simulink model "SIMULAZIONE_AF"  (R2020b)
settings: Solver=VariableStepAuto  StartTime=0.0  StopTime=10  RelTol=1e-3
libraries: simulink x1, dsparch4 x1
settings Model: Creator=danie  LastModifiedBy=danie

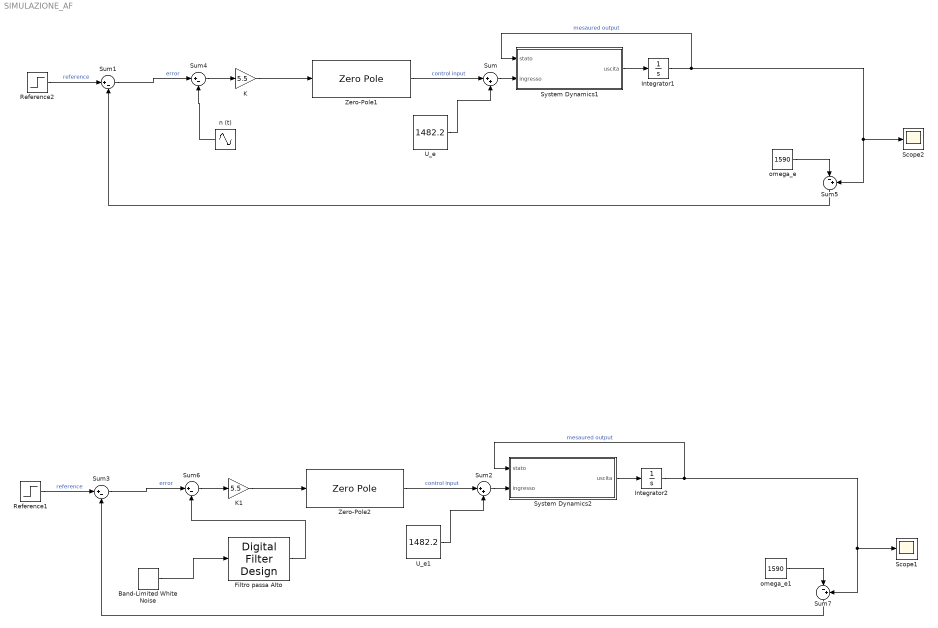
== system SIMULAZIONE_AF ==
  Band-Limited White Noise : simulink/Sources/Band-Limited White Noise  Cov=[500]  Ts=0.1  seed=[23341]
  Filtro passa Alto : dsparch4/Digital Filter Design  mwdsp_browser_bugfix_var=off
  Integrator1 : Integrator  InitialCondition=1590
  Integrator2 : Integrator  InitialCondition=1590
  K : Gain  Gain=5.5
  K1 : Gain  Gain=5.5
  Reference1 : Step  Time=0  After=4  SampleTime=0
  Reference2 : Step  Time=0  After=4  SampleTime=0
  Scope1 : Scope
  Scope2 : Scope
  Sum : Sum  Inputs=|++
  Sum{1,3..4,6} (4 alike) : Sum  Inputs=|+-
  Sum2 : Sum  Inputs=|++
  Sum5 : Sum  Inputs=|-+
  Sum7 : Sum  Inputs=|-+
  System Dynamics1 : MATLAB Function  TreatAsAtomicUnit=on
  System Dynamics2 : MATLAB Function  TreatAsAtomicUnit=on
  U_e : Constant  Value=1482.2
  U_e1 : Constant  Value=1482.2
  Zero-Pole1 : ZeroPole  Zeros=[-0.8192]  Poles=[0 -38.91]  Gain=[94.99]
  Zero-Pole2 : ZeroPole  Zeros=[-0.8192]  Poles=[0 -38.91]  Gain=[94.99]
  "n (t) " : Sin  Amplitude=0.025  Frequency=120  SampleTime=0
  omega_e : Constant  Value=1590
  omega_e1 : Constant  Value=1590
  wires:
  System Dynamics1/1(uscita) -> Integrator1/1
  "n (t) "/1 -> Sum4/2
  Integrator1/1 -> System Dynamics1/1(stato), Sum5/2, Scope2/1  "mesaured output"
  Reference2/1 -> Sum1/1  "reference"
  Sum1/1 -> Sum4/1  "error"
  Sum4/1 -> K/1
  Zero-Pole1/1 -> Sum/1  "control input"
  K/1 -> Zero-Pole1/1
  U_e/1 -> Sum/2
  Sum/1 -> System Dynamics1/2(ingresso)
  Sum5/1 -> Sum1/2
  omega_e/1 -> Sum5/1
  System Dynamics2/1(uscita) -> Integrator2/1
  U_e1/1 -> Sum2/2
  Zero-Pole2/1 -> Sum2/1  "control input"
  Sum7/1 -> Sum3/2
  Sum6/1 -> K1/1
  Reference1/1 -> Sum3/1  "reference"
  Integrator2/1 -> System Dynamics2/1(stato), Sum7/2, Scope1/1  "mesaured output"
  Sum3/1 -> Sum6/1  "error"
  Sum2/1 -> System Dynamics2/2(ingresso)
  K1/1 -> Zero-Pole2/1
  omega_e1/1 -> Sum7/1
  Filtro passa Alto/1 -> Sum6/2
  Band-Limited White Noise/1 -> Filtro passa Alto/1

== matlab function SIMULAZIONE_AF/System Dynamics1 ==
  data: stato input size=1; ingresso input size=1; uscita output size=1
function uscita  = systemDynamic(stato, ingresso)
stato_vero = stato;
ingresso_vero=ingresso;
beta = 0.3;
massa = 0.15;
e_i = 0.47;
inerzia = 0.75;
mu_d = 0.012;

uscita = (-beta*stato_vero - mu_d*massa*stato_vero*stato_vero*e_i*e_i + ingresso_vero)/(massa*e_i*e_i + inerzia ) ;

== matlab function SIMULAZIONE_AF/System Dynamics2 ==
  data: stato input size=1; ingresso input size=1; uscita output size=1
function uscita  = systemDynamic(stato, ingresso)
stato_vero = stato;
ingresso_vero=ingresso;
beta = 0.3;
massa = 0.15;
e_i = 0.47;
inerzia = 0.75;
mu_d = 0.012;

uscita = (-beta*stato_vero - mu_d*massa*stato_vero*stato_vero*e_i*e_i + ingresso_vero)/(massa*e_i*e_i + inerzia ) ;
